simulink model "HITL"  (R2020a)
settings: Solver=ode4  StartTime=0.0  StopTime=100  FixedStep=0.02  RelTol=1e-3  EnableMultiTasking=on
values from neighbouring files (symbols this model uses):
  g = data(5); Quad.b = data(6); Quad.d = data(7); Quad.l = data(8)    [Quad1.m]
undefined symbols (not defined in the file or in its folder): sigbuilder_block
libraries: aerolibutil x10, simulink x9, sharedutil x3, dspindex x2, dspmathops x2, vrlib x1
(part 1 of 2)
settings Model: Creator=Hisham  LastModifiedBy=Hisham
settings DataIOCC: ReturnWorkspaceOutputs=off
settings DebuggingCC: ArithmeticOperatorsInVariantConditions=warning
settings SFSimCC: SimUseLocalCustomCode=off  CustomCodeUndefinedFunction=UseInterfaceOnly
settings RTWCC: RTWUseLocalCustomCode=off
settings CodeAppCC: StateflowObjectComments=on

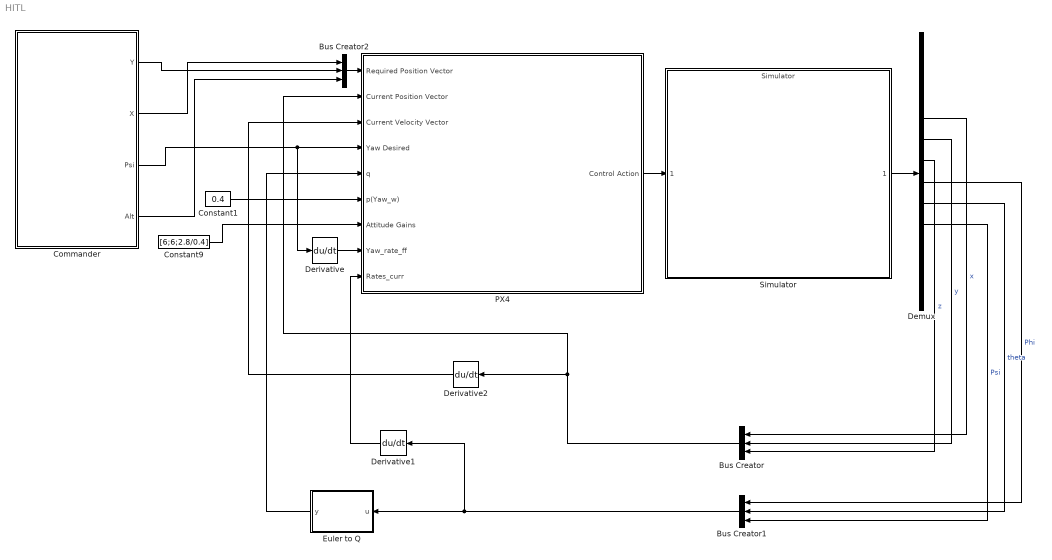
== system HITL ==
  Bus Creator : BusCreator  Inputs=3
  Bus Creator1 : BusCreator  Inputs=3
  Bus Creator2 : BusCreator  Inputs=3
  Commander : Subsystem
  Constant1 : Constant  Value=0.4
  Constant9 : Constant  Value=[6;6;2.8/0.4]
  Demux : Demux  Outputs=12
  Derivative : Derivative
  Derivative1 : Derivative
  Derivative2 : Derivative
  Euler to Q : MATLAB Function  TreatAsAtomicUnit=on
  PX4 : Subsystem
  Simulator : ModelReference  ModelNameDialog=Simulator.slx  SimulationMode=Normal  ModelReferenceVersion=1.27
  wires:
  Commander/2(X) -> Bus Creator2/1
  Commander/3(Psi) -> PX4/4(Yaw Desired), Derivative/1
  Commander/4(Alt) -> Bus Creator2/3
  PX4/1(Control Action) -> Simulator/1
  Demux/8 -> Bus Creator1/2  "theta"
  Demux/5 -> Bus Creator/2  "y"
  Demux/9 -> Bus Creator1/3  "Psi"
  Demux/7 -> Bus Creator1/1  "Phi"
  Demux/4 -> Bus Creator/1  "x"
  Demux/6 -> Bus Creator/3  "z"
  Simulator/1 -> Demux/1
  Bus Creator/1 -> PX4/2(Current Position Vector), Derivative2/1
  Bus Creator1/1 -> Derivative1/1, Euler to Q/1(u)
  Constant1/1 -> PX4/6(p(Yaw_w))
  Constant9/1 -> PX4/7(Attitude Gains)
  Commander/1(Y) -> Bus Creator2/2
  Bus Creator2/1 -> PX4/1(Required Position Vector)
  Derivative/1 -> PX4/8(Yaw_rate_ff)
  Derivative1/1 -> PX4/9(Rates_curr)
  Euler to Q/1(y) -> PX4/5(q)
  Derivative2/1 -> PX4/3(Current Velocity Vector)

== system HITL/Commander ==
  Alt_com : Constant  Value=-3
  Psi_com : Constant  Value=30*2*pi/180
  Signal Builder : Subsystem  Tag=STV Subsys  LoadFcn=sigbuilder_block('load');  StartFcn=sigbuilder_block('start');  StopFcn=sigbuilder_block('stop');  ClipboardFcn=sigbuilder_block('clipboard');  mask(Sigbuilder block){tuvar=[0:10]}
      mask help: Simulink:masks:SigbuilderBlock_MD
      mask init:
      | if ~strcmp(get_param(bdroot(gcbh),'SimulationStatus'),'stopped') tuvar = sigbuilder_block('maskInit'); end
      settings: CopyFcn=sigbuilder_block('copy');  DeleteFcn=sigbuilder_block('delete');  ModelCloseFcn=sigbuilder_block('modelClose');  PreSaveFcn=sigbuilder_block('preSave');  PauseFcn=sigbuilder_block('pause');  ContinueFcn=sigbuilder_block('continue');  NameChangeFcn=sigbuilder_block('namechange');  OpenFcn=sigbuilder_block('open',[6 30 1012.5 447.75 ]);  CloseFcn=sigbuilder_block('close');
      mask Display: plot(0, 0, 100, 100,[2, 2, 32, 32, 2], [68, 8, 8, 68, 68],[32, 2], [38, 38], [32, 19, 2],[53, 60, 44], [32, 17, 17, 2],[16, 16, 31, 31]);txt = getActiveGroup(gcbh);text(2, 100, txt,'verticalAlignment', 'top');
  X_com : Constant  Value=0
  Y_com : Constant  Value=0
  Y : Outport
  X : Outport  Port=2
  Psi : Outport  Port=3
  Alt : Outport  Port=4
  wires:
  Signal Builder/1(Y_com) -> Y/1
  Signal Builder/2(X_com) -> X/1
  Signal Builder/4(psi_com) -> Psi/1
  Signal Builder/3(alt_com) -> Alt/1

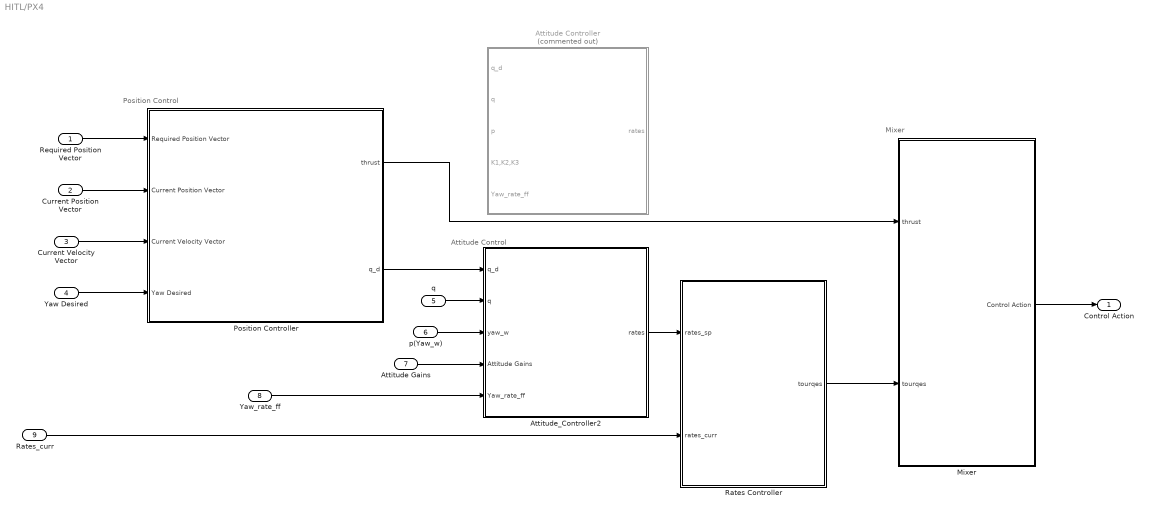
== system HITL/PX4 ==
  note: Mixer
  note: Position Control
  note: Attitude Control
  Required Position Vector : Inport
  Current Position Vector : Inport  Port=2
  Current Velocity Vector : Inport  Port=3
  Yaw Desired : Inport  Port=4
  q : Inport  Port=5
  p(Yaw_w) : Inport  Port=6
  Attitude Gains : Inport  Port=7
  Yaw_rate_ff : Inport  Port=8
  Rates_curr : Inport  Port=9
  Attitude Controller : Subsystem  Commented=on
  Attitude_Controller2 : Subsystem
  Mixer : Subsystem
  Position Controller : Subsystem
  Rates Controller : Subsystem
  Control Action : Outport
  wires:
  Rates_curr/1 -> Rates Controller/2(rates_curr)
  Attitude_Controller2/1(rates) -> Rates Controller/1(rates_sp)
  Mixer/1(Control Action) -> Control Action/1
  Rates Controller/1(tourqes) -> Mixer/2(tourqes)
  q/1 -> Attitude_Controller2/2(q)
  Attitude Gains/1 -> Attitude_Controller2/4(Attitude Gains)
  p(Yaw_w)/1 -> Attitude_Controller2/3(yaw_w)
  Yaw_rate_ff/1 -> Attitude_Controller2/5(Yaw_rate_ff)
  Position Controller/1(thrust) -> Mixer/1(thrust)
  Current Position Vector/1 -> Position Controller/2(Current Position Vector)
  Current Velocity Vector/1 -> Position Controller/3(Current Velocity Vector)
  Required Position Vector/1 -> Position Controller/1(Required Position Vector)
  Yaw Desired/1 -> Position Controller/4(Yaw Desired)
  Position Controller/2(q_d) -> Attitude_Controller2/1(q_d)

== system HITL/Commander/Signal Builder ==
  Demux : Demux  Tag=STV Demux
      settings: DisplayOption=none
  FromWs : FromWorkspace  Tag=STV FromWs  VariableName=tuvar
      SigBuilderData=|
      | common.afterFinalStr = 'Extrapolate'
      | common.sampleTime = 0
      | dataSet.timeRange = [0 60]
      | dataSet.name = 'Group 1'
      | sbobj.Groups.Name = 'Group 1'
      | sbobj.Groups.Signals(1).Name = 'Y_com'
      | sbobj.Groups.Signals(1).XData = [0 4 4 25 25 60]
      | sbobj.Groups.Signals(1).YData = [0 0 5 5 0 0]
      | sbobj.Groups.Signals(2).Name = 'X_com'
      | sbobj.Groups.Signals(2).XData = [0 12 12 42 42 60]
      | sbobj.Groups.Signals(2).YData = [0 0 5 5 0 0]
      | sbobj.Groups.Signals(3).Name = 'alt_com'
      | sbobj.Groups.Signals(3).XData = [0 10 10 60]
      | sbobj.Groups.Signals(3).YData = [1 1 5 5]
      | sbobj.Groups.Signals(4).Name = 'psi_com'
      | sbobj.Groups.Signals(4).XData = [0 1 60]
      | sbobj.Groups.Signals(4).YData = [0 0 0]
      | sbobj.Groups.TimeRange = [0 60]
  Y_com : Outport  Tag=STV Outport
  X_com : Outport  Tag=STV Outport  Port=2
  alt_com : Outport  Tag=STV Outport  Port=3
  psi_com : Outport  Tag=STV Outport  Port=4
  wires:
  FromWs/1 -> Demux/1
  Demux/1 -> Y_com/1
  Demux/2 -> X_com/1
  Demux/3 -> alt_com/1
  Demux/4 -> psi_com/1

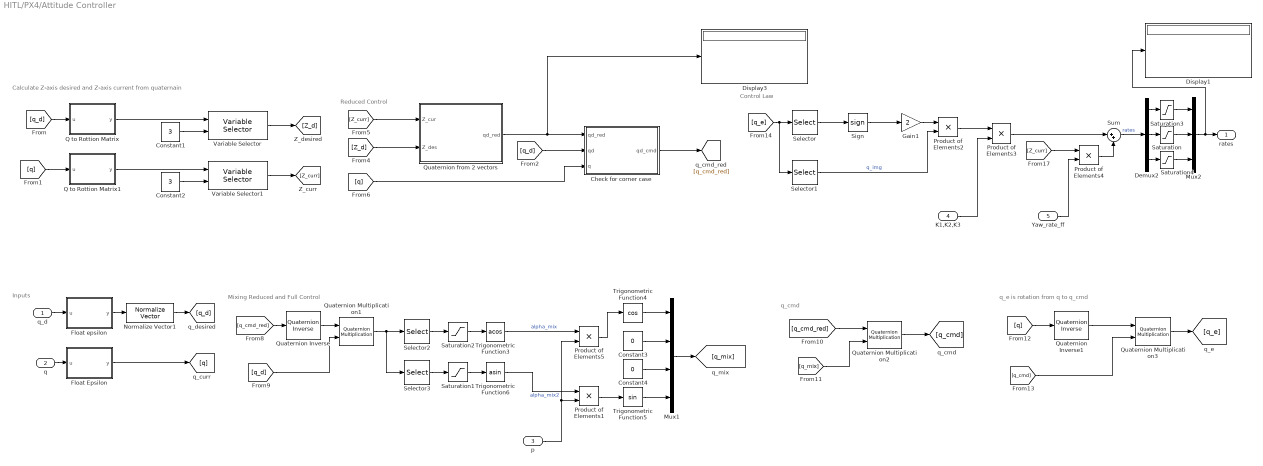
== system HITL/PX4/Attitude Controller ==
  note: Control Law
  note: q_e is rotation from q to q_cmd
  note: Inputs
  note: q_cmd
  note: Mixing Reduced and Full Control
  note: Reduced Control
  note: Calculate Z-axis desired and Z-axis current from quaternain
  q_d : Inport
  q : Inport  Port=2
  p : Inport  Port=3
  K1,K2,K3 : Inport  Port=4
  Yaw_rate_ff : Inport  Port=5
  Check for corner case : MATLAB Function  TreatAsAtomicUnit=on
  Constant1 : Constant  Value=3
  Constant2 : Constant  Value=3
  Constant3 : Constant  Value=0
  Constant4 : Constant  Value=0
  Demux2 : Demux  Outputs=3
  Display1 : Display
  Display3 : Display
  Float Epsilon : MATLAB Function  TreatAsAtomicUnit=on
  Float epsilon : MATLAB Function  TreatAsAtomicUnit=on
  Gain1 : Gain  Gain=2
  Mux1 : Mux
  Mux2 : Mux  Inputs=3
  Normalize Vector1 : vrlib/Utilities/Normalize Vector  maxzero=0
  Product of Elements{1..5} (5 alike) : Product  Inputs=**
  Q to Rottion Matrix : MATLAB Function  TreatAsAtomicUnit=on
  Q to Rottion Matrix1 : MATLAB Function  TreatAsAtomicUnit=on
  Quaternion Inverse : aerolibutil/Quaternion Inverse
  Quaternion Inverse1 : aerolibutil/Quaternion Inverse
  Quaternion Multiplication1 : aerolibutil/Quaternion Multiplication
  Quaternion Multiplication2 : aerolibutil/Quaternion Multiplication
  Quaternion Multiplication3 : aerolibutil/Quaternion Multiplication
  Quaternion from 2 vectors : MATLAB Function  TreatAsAtomicUnit=on
  Saturation : Saturate  UpperLimit=220*pi/180  LowerLimit=-220*pi/180
  Saturation1 : Saturate  UpperLimit=1  LowerLimit=-1
  Saturation2 : Saturate  UpperLimit=1  LowerLimit=-1
  Saturation3 : Saturate  UpperLimit=220*pi/180  LowerLimit=-220*pi/180
  Saturation4 : Saturate  UpperLimit=200*pi/180  LowerLimit=-200*pi/180
  Selector : Selector  InputPortWidth=4  IndexOptions=Index vector (dialog)  Indices=[1]  OutputSizes=1
  Selector1 : Selector  InputPortWidth=4  IndexOptions=Index vector (dialog)  Indices=[2 3 4]  OutputSizes=1
  Selector2 : Selector  InputPortWidth=4  IndexOptions=Index vector (dialog)  Indices=1  OutputSizes=1
  Selector3 : Selector  InputPortWidth=4  IndexOptions=Index vector (dialog)  Indices=4  OutputSizes=1
  Sign : Signum
  Sum : Sum  Inputs=|++
  Trigonometric Function3 : Trigonometry  Operator=acos
  Trigonometric Function4 : Trigonometry  Operator=cos
  Trigonometric Function5 : Trigonometry
  Trigonometric Function6 : Trigonometry  Operator=asin
  Variable Selector : dspindex/Variable Selector  NumInputs=1  rowsOrCols=Columns  IdxMode=Variable  Elements=[1 3]  ZerOneIdxMode=One-based  errmode=Clip Index  FillMode=on  FillValues=0
  Variable Selector1 : dspindex/Variable Selector  NumInputs=1  rowsOrCols=Columns  IdxMode=Variable  Elements=[1 3]  ZerOneIdxMode=One-based  errmode=Clip Index  FillMode=on  FillValues=0
  rates : Outport
  wires:
  Q to Rottion Matrix/1(y) -> Variable Selector/1
  Constant1/1 -> Variable Selector/2
  Q to Rottion Matrix1/1(y) -> Variable Selector1/1
  Constant2/1 -> Variable Selector1/2
  [q_d] -> Q to Rottion Matrix/1(u)
  [q] -> Q to Rottion Matrix1/1(u)
  Variable Selector/1 -> [Z_d]
  Variable Selector1/1 -> [Z_curr]
  [q] -> Check for corner case/3(q)
  Check for corner case/1(qd_cmd) -> [q_cmd_red]
  [q_cmd_red] -> Quaternion Inverse/1
  Quaternion Inverse/1 -> Quaternion Multiplication1/1
  [q_d] -> Quaternion Multiplication1/2
  [q_cmd_red] -> Quaternion Multiplication2/1
  [q_mix] -> Quaternion Multiplication2/2
  Quaternion Multiplication2/1 -> [q_cmd]
  [q] -> Quaternion Inverse1/1
  Quaternion Inverse1/1 -> Quaternion Multiplication3/1
  [q_cmd] -> Quaternion Multiplication3/2
  Quaternion Multiplication3/1 -> [q_e]
  [q_e] -> Selector1/1, Selector/1
  Selector/1 -> Sign/1
  Sign/1 -> Gain1/1
  Gain1/1 -> Product of Elements2/1
  Selector1/1 -> Product of Elements2/2  "q_img"
  Product of Elements2/1 -> Product of Elements3/1
  Product of Elements3/1 -> Sum/1
  [Z_curr] -> Product of Elements4/1
  Product of Elements4/1 -> Sum/2
  Selector2/1 -> Saturation2/1
  Trigonometric Function3/1 -> Product of Elements5/1  "alpha_mix"
  Product of Elements5/1 -> Trigonometric Function4/1
  Trigonometric Function5/1 -> Mux1/4
  Constant4/1 -> Mux1/3
  Constant3/1 -> Mux1/2
  Trigonometric Function4/1 -> Mux1/1
  Mux1/1 -> [q_mix]
  q_d/1 -> Float epsilon/1(u)
  Normalize Vector1/1 -> [q_d]
  Float Epsilon/1(y) -> [q]
  q/1 -> Float Epsilon/1(u)
  Float epsilon/1(y) -> Normalize Vector1/1
  Mux2/1 -> Display1/1, rates/1
  [Z_d] -> Quaternion from 2 vectors/2(Z_des)
  Quaternion from 2 vectors/1(qd_red) -> Display3/1, Check for corner case/1(qd_red)
  [Z_curr] -> Quaternion from 2 vectors/1(Z_cur)
  Demux2/2 -> Saturation/1
  Demux2/3 -> Saturation4/1
  Saturation/1 -> Mux2/2
  Saturation3/1 -> Mux2/1
  Demux2/1 -> Saturation3/1
  Sum/1 -> Demux2/1  "rates"
  Saturation4/1 -> Mux2/3
  [q_d] -> Check for corner case/2(qd)
  Quaternion Multiplication1/1 -> Selector3/1, Selector2/1
  Saturation2/1 -> Trigonometric Function3/1
  K1,K2,K3/1 -> Product of Elements3/2
  Yaw_rate_ff/1 -> Product of Elements4/2
  p/1 -> Product of Elements1/2, Product of Elements5/2
  Saturation1/1 -> Trigonometric Function6/1
  Selector3/1 -> Saturation1/1
  Product of Elements1/1 -> Trigonometric Function5/1
  Trigonometric Function6/1 -> Product of Elements1/1  "alpha_mix2"

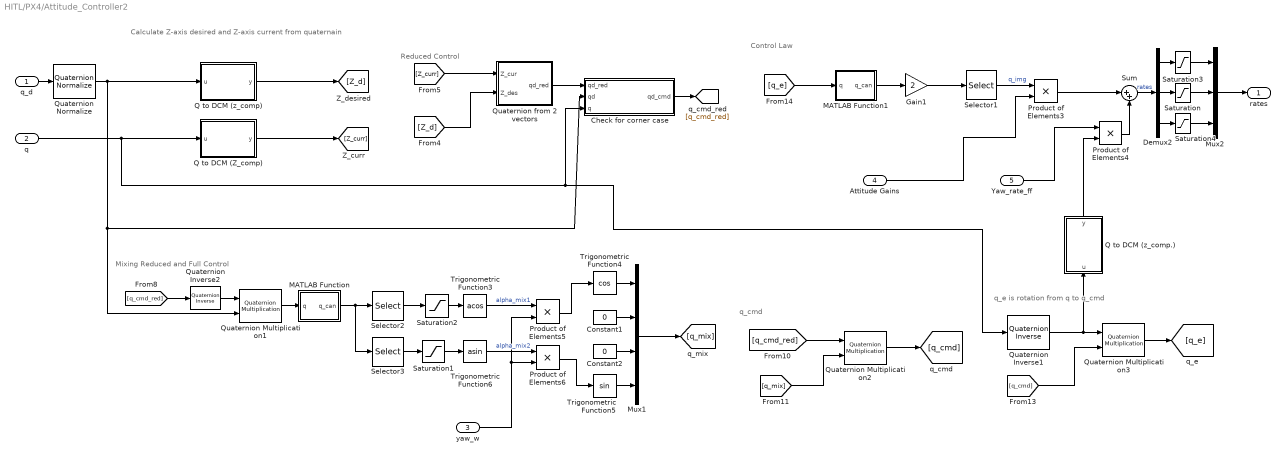
== system HITL/PX4/Attitude_Controller2 ==
  note: Mixing Reduced and Full Control
  note: Calculate Z-axis desired and Z-axis current from quaternain
  note: Control Law
  note: Reduced Control
  note: q_cmd
  note: q_e is rotation from q to q_cmd
  q_d : Inport
  q : Inport  Port=2
  yaw_w : Inport  Port=3
  Attitude Gains : Inport  Port=4
  Yaw_rate_ff : Inport  Port=5
  Check for corner case : MATLAB Function  TreatAsAtomicUnit=on
  Constant1 : Constant  Value=0
  Constant2 : Constant  Value=0
  Demux2 : Demux  Outputs=3
  Gain1 : Gain  Gain=2
  MATLAB Function : MATLAB Function  TreatAsAtomicUnit=on
  MATLAB Function1 : MATLAB Function  TreatAsAtomicUnit=on
  Mux1 : Mux
  Mux2 : Mux  Inputs=3
  Product of Elements{3..6} (4 alike) : Product  Inputs=**
  Q to DCM (Z_comp) : MATLAB Function  TreatAsAtomicUnit=on
  Q to DCM (z_comp) : MATLAB Function  TreatAsAtomicUnit=on
  Q to DCM (z_comp.) : MATLAB Function  TreatAsAtomicUnit=on
  Quaternion Inverse1 : aerolibutil/Quaternion Inverse
  Quaternion Inverse2 : aerolibutil/Quaternion Inverse
  Quaternion Multiplication1 : aerolibutil/Quaternion Multiplication
  Quaternion Multiplication2 : aerolibutil/Quaternion Multiplication
  Quaternion Multiplication3 : aerolibutil/Quaternion Multiplication
  Quaternion Normalize : sharedutil/Quaternion Normalize  aMode=aMode
      settings: SourceProductBaseCode=AE,PW,MT,VE,VP
  Quaternion from 2 vectors : MATLAB Function  TreatAsAtomicUnit=on
  Saturation : Saturate  UpperLimit=220*pi/180  LowerLimit=-220*pi/180
  Saturation1 : Saturate  UpperLimit=1  LowerLimit=-1
  Saturation2 : Saturate  UpperLimit=1  LowerLimit=-1
  Saturation3 : Saturate  UpperLimit=220*pi/180  LowerLimit=-220*pi/180
  Saturation4 : Saturate  UpperLimit=200*pi/180  LowerLimit=-200*pi/180
  Selector1 : Selector  InputPortWidth=4  IndexOptions=Index vector (dialog)  Indices=[2 3 4]  OutputSizes=1
  Selector2 : Selector  InputPortWidth=4  IndexOptions=Index vector (dialog)  Indices=1  OutputSizes=1
  Selector3 : Selector  InputPortWidth=4  IndexOptions=Index vector (dialog)  Indices=4  OutputSizes=1
  Sum : Sum  Inputs=|++
  Trigonometric Function3 : Trigonometry  Operator=acos
  Trigonometric Function4 : Trigonometry  Operator=cos
  Trigonometric Function5 : Trigonometry
  Trigonometric Function6 : Trigonometry  Operator=asin
  rates : Outport
  wires:
  Mux2/1 -> rates/1
  Saturation3/1 -> Mux2/1
  Saturation4/1 -> Mux2/3
  Saturation/1 -> Mux2/2
  Demux2/3 -> Saturation4/1
  Demux2/1 -> Saturation3/1
  Demux2/2 -> Saturation/1
  Sum/1 -> Demux2/1  "rates"
  [Z_d] -> Quaternion from 2 vectors/2(Z_des)
  Quaternion from 2 vectors/1(qd_red) -> Check for corner case/1(qd_red)
  [Z_curr] -> Quaternion from 2 vectors/1(Z_cur)
  MATLAB Function1/1(q_can) -> Gain1/1
  [q_e] -> MATLAB Function1/1(q)
  Gain1/1 -> Selector1/1
  Selector1/1 -> Product of Elements3/1  "q_img"
  Check for corner case/1(qd_cmd) -> [q_cmd_red]
  q/1 -> Q to DCM (Z_comp)/1(u), Quaternion Inverse1/1, Check for corner case/3(q)
  Quaternion Normalize/1 -> Q to DCM (z_comp)/1(u), Check for corner case/2(qd), Quaternion Multiplication1/2
  MATLAB Function/1(q_can) -> Selector2/1, Selector3/1
  Quaternion Multiplication1/1 -> MATLAB Function/1(q)
  q_d/1 -> Quaternion Normalize/1
  Quaternion Inverse2/1 -> Quaternion Multiplication1/1
  [q_cmd_red] -> Quaternion Inverse2/1
  Mux1/1 -> [q_mix]
  Quaternion Inverse1/1 -> Q to DCM (z_comp.)/1(u), Quaternion Multiplication3/1
  Product of Elements3/1 -> Sum/1
  [q_cmd] -> Quaternion Multiplication3/2
  [q_mix] -> Quaternion Multiplication2/2
  [q_cmd_red] -> Quaternion Multiplication2/1
  Selector2/1 -> Saturation2/1
  Quaternion Multiplication3/1 -> [q_e]
  Selector3/1 -> Saturation1/1
  Yaw_rate_ff/1 -> Product of Elements4/1
  Product of Elements4/1 -> Sum/2
  Saturation2/1 -> Trigonometric Function3/1
  Trigonometric Function3/1 -> Product of Elements5/1  "alpha_mix1"
  Quaternion Multiplication2/1 -> [q_cmd]
  Q to DCM (z_comp.)/1(y) -> Product of Elements4/2
  Trigonometric Function4/1 -> Mux1/1
  Product of Elements5/1 -> Trigonometric Function4/1
  Trigonometric Function5/1 -> Mux1/4
  Trigonometric Function6/1 -> Product of Elements6/1  "alpha_mix2"
  Product of Elements6/1 -> Trigonometric Function5/1
  Saturation1/1 -> Trigonometric Function6/1
  Q to DCM (z_comp)/1(y) -> [Z_d]
  Q to DCM (Z_comp)/1(y) -> [Z_curr]
  yaw_w/1 -> Product of Elements5/2, Product of Elements6/2
  Attitude Gains/1 -> Product of Elements3/2
  Constant1/1 -> Mux1/2
  Constant2/1 -> Mux1/3

== system HITL/PX4/Mixer ==
  thrust : Inport
  tourqes : Inport  Port=2
  Display : Display
  "Float Epsilon " : MATLAB Function
  Gain : Gain  Gain=-1
  Iris mixer : Constant  Value=[-0.4377 0.7071 -0.9091 -1; 0.4377 -0.7071 -1 -1; 0.4377 0.7071 0.9091 -1;-0.4377 -0.7071 1 -1]
  Length : MATLABFcn  MATLABFcn=norm
  Mux : Mux  Inputs=2
  Quad_x mixer : Constant  Value=[-0.7071 0.7071 1 -1; 0.7071 -0.7071 1 -1; 0.7071 0.7071 -1 -1;-0.7071 -0.7071 -1 -1]
  Control Action : Outport
  wires:
  thrust/1 -> Length/1
  tourqes/1 -> Mux/1
  Length/1 -> Gain/1
  Mux/1 -> "Float Epsilon "/1(u)
  Gain/1 -> Mux/2
  "Float Epsilon "/1(y) -> Control Action/1, Display/1

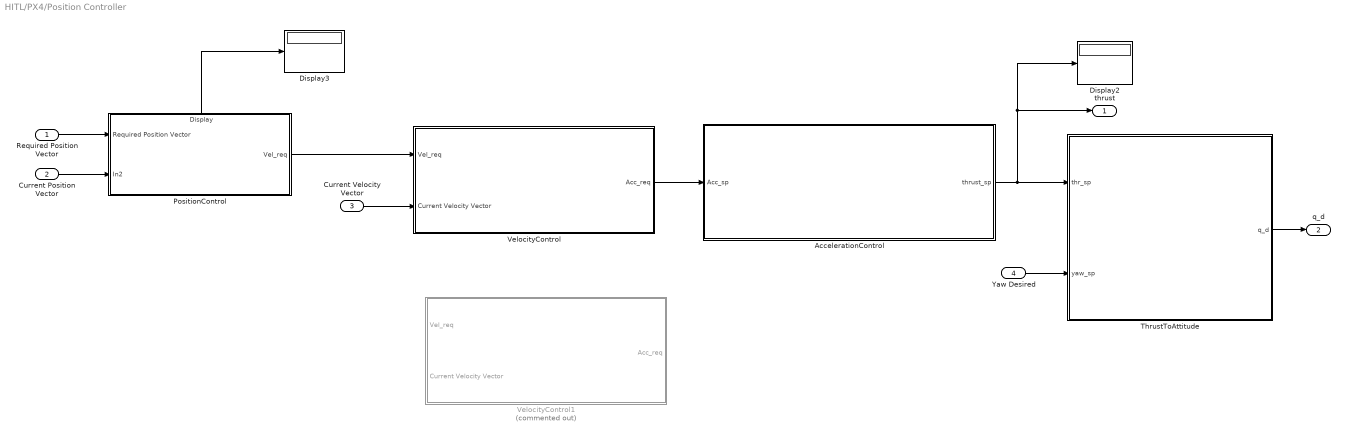
== system HITL/PX4/Position Controller ==
  Required Position Vector : Inport
  Current Position Vector : Inport  Port=2
  Current Velocity Vector : Inport  Port=3
  Yaw Desired : Inport  Port=4
  AccelerationControl : Subsystem
  Display2 : Display
  Display3 : Display
  PositionControl : Subsystem
      settings: PortSchema="{\"entries\":[{\"content\":{\"sides\":[{\"content\":{\"connectorIds\":[\"In1\",\"In2\"]},\"type\":\"ConnectorPlacement.EquallySpacedRectSide\",\"uuid\":\"a4ba3283-86cb-408b-aae8-413f3026a3b7\"},{\"content\":{\"connectorIds\":[\"Out1\"],\"side\":\"RIGHT\"},\"type\":\"ConnectorPlacement.EquallySpacedRectSide\",\"uuid\":\"45b02b29-05a1-4a67-8748-9d19bb26d9bb\"},{\"content\":{\"connectorIds\":[\"Out2\"],\"side\":\"TOP\"},\"type\":\"ConnectorPlacement.EquallySpacedRectSide\",\"uuid\":\"6a5eeb60-33a1-4be7-a33c-7d288ab8de61\"}]},\"type\":\"ConnectorPlacement.EquallySpacedConnector\",\"uuid\":\"25cb5f3a-4277-4784-9d46-e5c601df25b2\"}],\"packageUris\":[\"http://schema.mathworks.com/mf0/Connector/19700101\"],\"version\":\"1.0\"}"
  ThrustToAttitude : Subsystem
  VelocityControl : Subsystem
  VelocityControl1 : Subsystem  Commented=on
  thrust : Outport
  q_d : Outport  Port=2
  wires:
  Required Position Vector/1 -> PositionControl/1(Required Position Vector)
  Current Position Vector/1 -> PositionControl/2(In2)
  PositionControl/2(Display) -> Display3/1
  PositionControl/1(Vel_req) -> VelocityControl/1(Vel_req)
  Current Velocity Vector/1 -> VelocityControl/2(Current Velocity Vector)
  AccelerationControl/1(thrust_sp) -> Display2/1, thrust/1, ThrustToAttitude/1(thr_sp)
  VelocityControl/1(Acc_req) -> AccelerationControl/1(Acc_sp)
  ThrustToAttitude/1(q_d) -> q_d/1
  Yaw Desired/1 -> ThrustToAttitude/2(yaw_sp)

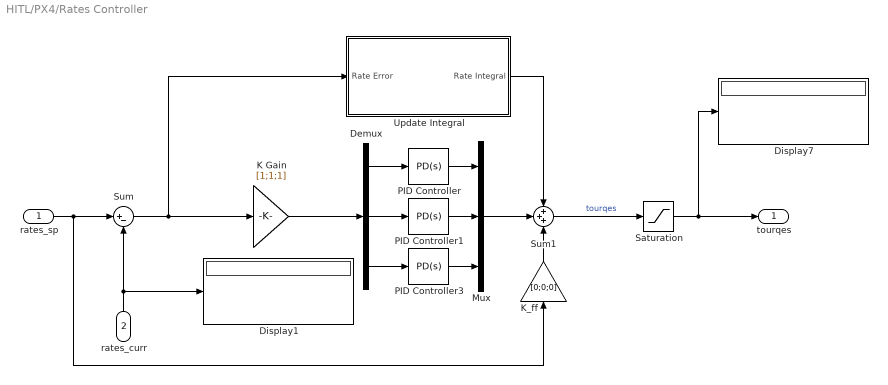
== system HITL/PX4/Rates Controller ==
  rates_sp : Inport
  rates_curr : Inport  Port=2
  Demux : Demux  Outputs=3
  Display1 : Display
  Display7 : Display
  K Gain : Gain  Gain=[1;1;1]
  K_ff : Gain  Gain=[0;0;0]
  Mux : Mux  Inputs=3
  PID Controller : simulink/Continuous/PID Controller  Controller=PD  Form=Parallel  TimeDomain=Continuous-time  UseExternalTs=off  SampleTime=-1  IntegratorMethod=Forward Euler  FilterMethod=Forward Euler  ControllerParametersSource=internal  P=0.2  I=0.2  D=-0.003  UseFilter=on  N=100  TunerSelectOption=Transfer Function Based (PID Tuner App)  InitialConditionSource=internal  InitialConditionForIntegrator=0  InitialConditionForFilter=0  DifferentiatorICPrevScaledInput=0  ExternalReset=none  TrackingMode=off  Kt=1  LimitOutput=off  UpperSaturationLimit=inf  LowerSaturationLimit=-inf  LinearizeAsGain=on  AntiWindupMode=none  Kb=1  POutMin=[]  POutMax=[]  IOutMin=[]  IOutMax=[]  DOutMin=[]  DOutMax=[]  NOutMin=[]  NOutMax=[]  SumOutMin=[]  SumOutMax=[]  SaturationOutMin=[]  SaturationOutMax=[]  PParamMin=[]  PParamMax=[]  IParamMin=[]  IParamMax=[]  DParamMin=[]  DParamMax=[]  NParamMin=[]  NParamMax=[]  KbParamMin=[]  KbParamMax=[]  KtParamMin=[]  KtParamMax=[]  KbOutMin=[]  KbOutMax=[]  KtOutMin=[]  KtOutMax=[]  IntegratorOutMin=[]  IntegratorOutMax=[]  FilterOutMin=[]  FilterOutMax=[]  SumI1OutMin=[]  SumI1OutMax=[]  SumI2OutMin=[]  SumI2OutMax=[]  SumI3OutMin=[]  SumI3OutMax=[]  SumI4OutMin=[]  SumI4OutMax=[]  SumDOutMin=[]  SumDOutMax=[]  DifferentiatorOutMin=[]  DifferentiatorOutMax=[]  FilterDiffOutCoefMin=[]  FilterDiffOutCoefMax=[]  ReciprocalOutMin=[]  ReciprocalOutMax=[]  SumDenOutMin=[]  SumDenOutMax=[]  SumNumOutMin=[]  SumNumOutMax=[]  DivideOutMin=[]  DivideOutMax=[]  UdiffTsProdOutMin=[]  UdiffTsProdOutMax=[]  NTsProdOutMin=[]  NTsProdOutMax=[]  UintegralTsProdOutMin=[]  UintegralTsProdOutMax=[]  UngainTsProdOutMin=[]  UngainTsProdOutMax=[]  IntegratorContinuousStateAttributes=''  IntegratorStateMustResolveToSignalObject=off  IntegratorRTWStateStorageClass=Auto  FilterContinuousStateAttributes=''  FilterStateMustResolveToSignalObject=off  FilterRTWStateStorageClass=Auto  ParallelPVariant=InternalParameters  IdealPVariant=Disabled  IVariant=Disabled  DVariant=InternalParameters  IntegratorVariant=Disabled  SatVariant=Disabled  AWVariant=Disabled  PCopyVariant=Disabled  TRVariant=Disabled  FdbkBlocksVariant=Forward  IdealPFdbkVariant=Disabled  SatFdbkVariant=Disabled  DerivativeFilterVariant=ContFilter  NVariant=InternalParameters  NCopyVariant=Disabled  FilterICVariant=InternalICsFilter  IntegratorICVariant=Disabled  ExternalResetVariant=Disabled  TRSumVariant=Passthrough  SumFdbkVariant=Disabled  SumVariant=Sum_PD  TsampFilterVariant=InternalTs  TsampNgainVariant=Passthrough  TsampIntegralVariant=Disabled_SignalSpec
  PID Controller1 : simulink/Continuous/PID Controller  Controller=PD  Form=Parallel  TimeDomain=Continuous-time  UseExternalTs=off  SampleTime=-1  IntegratorMethod=Forward Euler  FilterMethod=Forward Euler  ControllerParametersSource=internal  P=0.2  I=0.2  D=-0.003  UseFilter=on  N=100  TunerSelectOption=Transfer Function Based (PID Tuner App)  InitialConditionSource=internal  InitialConditionForIntegrator=0  InitialConditionForFilter=0  DifferentiatorICPrevScaledInput=0  ExternalReset=none  TrackingMode=off  Kt=1  LimitOutput=off  UpperSaturationLimit=inf  LowerSaturationLimit=-inf  LinearizeAsGain=on  AntiWindupMode=none  Kb=1  POutMin=[]  POutMax=[]  IOutMin=[]  IOutMax=[]  DOutMin=[]  DOutMax=[]  NOutMin=[]  NOutMax=[]  SumOutMin=[]  SumOutMax=[]  SaturationOutMin=[]  SaturationOutMax=[]  PParamMin=[]  PParamMax=[]  IParamMin=[]  IParamMax=[]  DParamMin=[]  DParamMax=[]  NParamMin=[]  NParamMax=[]  KbParamMin=[]  KbParamMax=[]  KtParamMin=[]  KtParamMax=[]  KbOutMin=[]  KbOutMax=[]  KtOutMin=[]  KtOutMax=[]  IntegratorOutMin=[]  IntegratorOutMax=[]  FilterOutMin=[]  FilterOutMax=[]  SumI1OutMin=[]  SumI1OutMax=[]  SumI2OutMin=[]  SumI2OutMax=[]  SumI3OutMin=[]  SumI3OutMax=[]  SumI4OutMin=[]  SumI4OutMax=[]  SumDOutMin=[]  SumDOutMax=[]  DifferentiatorOutMin=[]  DifferentiatorOutMax=[]  FilterDiffOutCoefMin=[]  FilterDiffOutCoefMax=[]  ReciprocalOutMin=[]  ReciprocalOutMax=[]  SumDenOutMin=[]  SumDenOutMax=[]  SumNumOutMin=[]  SumNumOutMax=[]  DivideOutMin=[]  DivideOutMax=[]  UdiffTsProdOutMin=[]  UdiffTsProdOutMax=[]  NTsProdOutMin=[]  NTsProdOutMax=[]  UintegralTsProdOutMin=[]  UintegralTsProdOutMax=[]  UngainTsProdOutMin=[]  UngainTsProdOutMax=[]  IntegratorContinuousStateAttributes=''  IntegratorStateMustResolveToSignalObject=off  IntegratorRTWStateStorageClass=Auto  FilterContinuousStateAttributes=''  FilterStateMustResolveToSignalObject=off  FilterRTWStateStorageClass=Auto  ParallelPVariant=InternalParameters  IdealPVariant=Disabled  IVariant=Disabled  DVariant=InternalParameters  IntegratorVariant=Disabled  SatVariant=Disabled  AWVariant=Disabled  PCopyVariant=Disabled  TRVariant=Disabled  FdbkBlocksVariant=Forward  IdealPFdbkVariant=Disabled  SatFdbkVariant=Disabled  DerivativeFilterVariant=ContFilter  NVariant=InternalParameters  NCopyVariant=Disabled  FilterICVariant=InternalICsFilter  IntegratorICVariant=Disabled  ExternalResetVariant=Disabled  TRSumVariant=Passthrough  SumFdbkVariant=Disabled  SumVariant=Sum_PD  TsampFilterVariant=InternalTs  TsampNgainVariant=Passthrough  TsampIntegralVariant=Disabled_SignalSpec
  PID Controller3 : simulink/Continuous/PID Controller  Controller=PD  Form=Parallel  TimeDomain=Continuous-time  UseExternalTs=off  SampleTime=-1  IntegratorMethod=Forward Euler  FilterMethod=Forward Euler  ControllerParametersSource=internal  P=0.2  I=0.1  D=0  UseFilter=on  N=100  TunerSelectOption=Transfer Function Based (PID Tuner App)  InitialConditionSource=internal  InitialConditionForIntegrator=0  InitialConditionForFilter=0  DifferentiatorICPrevScaledInput=0  ExternalReset=none  TrackingMode=off  Kt=1  LimitOutput=off  UpperSaturationLimit=inf  LowerSaturationLimit=-inf  LinearizeAsGain=on  AntiWindupMode=none  Kb=1  POutMin=[]  POutMax=[]  IOutMin=[]  IOutMax=[]  DOutMin=[]  DOutMax=[]  NOutMin=[]  NOutMax=[]  SumOutMin=[]  SumOutMax=[]  SaturationOutMin=[]  SaturationOutMax=[]  PParamMin=[]  PParamMax=[]  IParamMin=[]  IParamMax=[]  DParamMin=[]  DParamMax=[]  NParamMin=[]  NParamMax=[]  KbParamMin=[]  KbParamMax=[]  KtParamMin=[]  KtParamMax=[]  KbOutMin=[]  KbOutMax=[]  KtOutMin=[]  KtOutMax=[]  IntegratorOutMin=[]  IntegratorOutMax=[]  FilterOutMin=[]  FilterOutMax=[]  SumI1OutMin=[]  SumI1OutMax=[]  SumI2OutMin=[]  SumI2OutMax=[]  SumI3OutMin=[]  SumI3OutMax=[]  SumI4OutMin=[]  SumI4OutMax=[]  SumDOutMin=[]  SumDOutMax=[]  DifferentiatorOutMin=[]  DifferentiatorOutMax=[]  FilterDiffOutCoefMin=[]  FilterDiffOutCoefMax=[]  ReciprocalOutMin=[]  ReciprocalOutMax=[]  SumDenOutMin=[]  SumDenOutMax=[]  SumNumOutMin=[]  SumNumOutMax=[]  DivideOutMin=[]  DivideOutMax=[]  UdiffTsProdOutMin=[]  UdiffTsProdOutMax=[]  NTsProdOutMin=[]  NTsProdOutMax=[]  UintegralTsProdOutMin=[]  UintegralTsProdOutMax=[]  UngainTsProdOutMin=[]  UngainTsProdOutMax=[]  IntegratorContinuousStateAttributes=''  IntegratorStateMustResolveToSignalObject=off  IntegratorRTWStateStorageClass=Auto  FilterContinuousStateAttributes=''  FilterStateMustResolveToSignalObject=off  FilterRTWStateStorageClass=Auto  ParallelPVariant=InternalParameters  IdealPVariant=Disabled  IVariant=Disabled  DVariant=InternalParameters  IntegratorVariant=Disabled  SatVariant=Disabled  AWVariant=Disabled  PCopyVariant=Disabled  TRVariant=Disabled  FdbkBlocksVariant=Forward  IdealPFdbkVariant=Disabled  SatFdbkVariant=Disabled  DerivativeFilterVariant=ContFilter  NVariant=InternalParameters  NCopyVariant=Disabled  FilterICVariant=InternalICsFilter  IntegratorICVariant=Disabled  ExternalResetVariant=Disabled  TRSumVariant=Passthrough  SumFdbkVariant=Disabled  SumVariant=Sum_PD  TsampFilterVariant=InternalTs  TsampNgainVariant=Passthrough  TsampIntegralVariant=Disabled_SignalSpec
  Saturation : Saturate  UpperLimit=1  LowerLimit=-1
  Sum : Sum  Inputs=|+-
  Sum1 : Sum  Inputs=+++
  Update Integral : Subsystem
  tourqes : Outport
  wires:
  Sum1/1 -> Saturation/1  "tourqes"
  Sum/1 -> Update Integral/1(Rate Error), K Gain/1
  Demux/3 -> PID Controller3/1
  Demux/2 -> PID Controller1/1
  Demux/1 -> PID Controller/1
  PID Controller1/1 -> Mux/2
  PID Controller/1 -> Mux/1
  Saturation/1 -> Display7/1, tourqes/1
  PID Controller3/1 -> Mux/3
  K Gain/1 -> Demux/1
  rates_sp/1 -> K_ff/1, Sum/1
  Mux/1 -> Sum1/2
  K_ff/1 -> Sum1/3
  Update Integral/1(Rate Integral) -> Sum1/1
  rates_curr/1 -> Display1/1, Sum/2

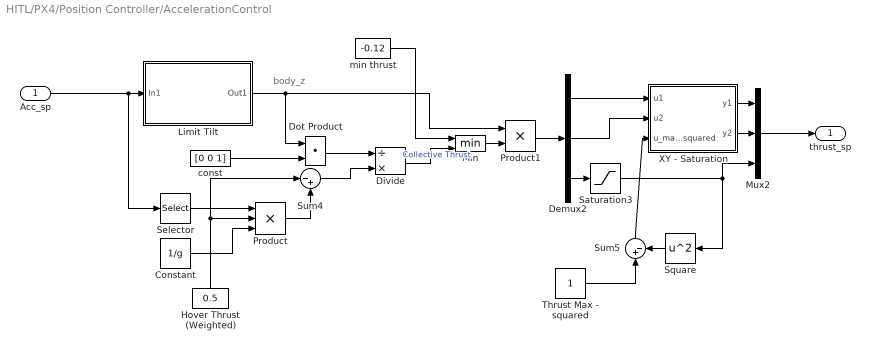
== system HITL/PX4/Position Controller/AccelerationControl ==
  note: body_z
  Acc_sp : Inport
  Constant : Constant  Value=1/g
  Demux2 : Demux  Outputs=3
  Divide : Product  Inputs=/*
  Dot Product : DotProduct  InputSameDT=on  OutDataTypeStr=Inherit: Inherit via internal rule
  Hover Thrust (Weighted) : Constant  Value=0.5
  Limit Tilt : Subsystem
  Min : MinMax  Inputs=2
  Mux2 : Mux  Inputs=3
  Product : Product  Inputs=3
  Product1 : Product
  Saturation3 : Saturate  UpperLimit=0  LowerLimit=-1
  Selector : Selector  InputPortWidth=3  IndexOptions=Index vector (dialog)  Indices=[3]  OutputSizes=1
  Square : Math  Operator=square  SaturateOnIntegerOverflow=on
  Sum4 : Sum  Inputs=|-+
  Sum5 : Sum  Inputs=|+-
  Thrust Max - squared : Constant
  XY - Saturation : MATLAB Function  TreatAsAtomicUnit=on
  const : Constant  Value=[0 0 1]
  min thrust : Constant  Value=-0.12
  thrust_sp : Outport
  wires:
  Limit Tilt/1(Out1) -> Product1/1, Dot Product/1
  Selector/1 -> Product/1
  Acc_sp/1 -> Selector/1, Limit Tilt/1(In1)
  Square/1 -> Sum5/2
  Saturation3/1 -> Mux2/3, Square/1
  Demux2/2 -> XY - Saturation/2(u2)
  Constant/1 -> Product/3
  XY - Saturation/2(y2) -> Mux2/2
  Hover Thrust (Weighted)/1 -> Product/2, Sum4/1
  XY - Saturation/1(y1) -> Mux2/1
  Demux2/1 -> XY - Saturation/1(u1)
  Demux2/3 -> Saturation3/1
  min thrust/1 -> Min/1
  Dot Product/1 -> Divide/1
  Product/1 -> Sum4/2
  const/1 -> Dot Product/2
  Product1/1 -> Demux2/1
  Sum4/1 -> Divide/2
  Min/1 -> Product1/2
  Thrust Max - squared/1 -> Sum5/1
  Divide/1 -> Min/2  "Collective Thrust"
  Sum5/1 -> XY - Saturation/3(u_max_squared)
  Mux2/1 -> thrust_sp/1

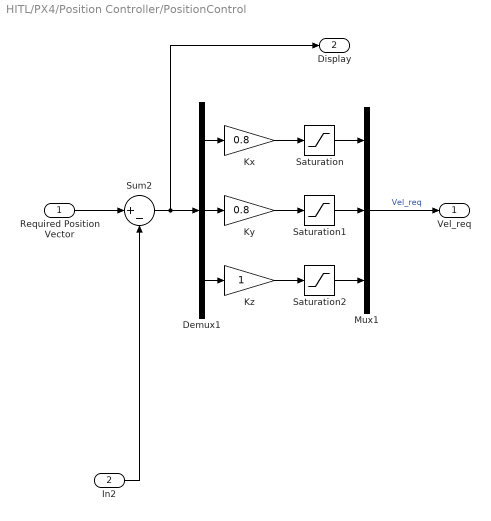
== system HITL/PX4/Position Controller/PositionControl ==
  Required Position Vector : Inport
  In2 : Inport  Port=2
  Demux1 : Demux  Outputs=3
  Kx : Gain  Gain=0.8
  Ky : Gain  Gain=0.8
  Kz : Gain
  Mux1 : Mux  Inputs=3
  Saturation : Saturate  UpperLimit=12  LowerLimit=-12
  Saturation1 : Saturate  UpperLimit=12  LowerLimit=-12
  Saturation2 : Saturate  UpperLimit=1  LowerLimit=-3
  Sum2 : Sum  Inputs=|+-
  Vel_req : Outport
  Display : Outport  Port=2
  wires:
  Demux1/3 -> Kz/1
  Demux1/2 -> Ky/1
  Saturation1/1 -> Mux1/2
  Kx/1 -> Saturation/1
  Required Position Vector/1 -> Sum2/1
  Demux1/1 -> Kx/1
  Saturation/1 -> Mux1/1
  Ky/1 -> Saturation1/1
  Sum2/1 -> Display/1, Demux1/1
  Saturation2/1 -> Mux1/3
  Kz/1 -> Saturation2/1
  In2/1 -> Sum2/2
  Mux1/1 -> Vel_req/1  "Vel_req"

== system HITL/PX4/Position Controller/ThrustToAttitude ==
  thr_sp : Inport
  yaw_sp : Inport  Port=2
  Matrix Concatenate : Concatenate  NumInputs=3  Mode=Multidimensional array  ConcatenateDimension=2
  Rotaion Matrix To Q : MATLAB Function  TreatAsAtomicUnit=on
  Thrust To Attitude : Subsystem
  q_d : Outport
  wires:
  Thrust To Attitude/3(Rz) -> Matrix Concatenate/3
  Matrix Concatenate/1 -> Rotaion Matrix To Q/1(u)  "R_sp"
  Thrust To Attitude/1(Rx) -> Matrix Concatenate/1
  Thrust To Attitude/2(Ry) -> Matrix Concatenate/2
  Rotaion Matrix To Q/1(y) -> q_d/1  "q_d"
  thr_sp/1 -> Thrust To Attitude/1(thr_sp)
  yaw_sp/1 -> Thrust To Attitude/2(yaw_sp)

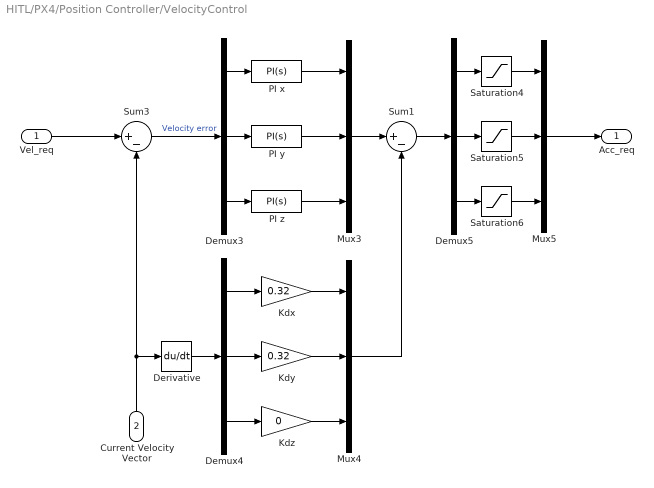
== system HITL/PX4/Position Controller/VelocityControl ==
  Vel_req : Inport
  Current Velocity Vector : Inport  Port=2
  Demux3 : Demux  Outputs=3
  Demux4 : Demux  Outputs=3
  Demux5 : Demux  Outputs=3
  Derivative : Derivative
  Kdx : Gain  Gain=0.32
  Kdy : Gain  Gain=0.32
  Kdz : Gain  Gain=0
  Mux3 : Mux  Inputs=3
  Mux4 : Mux  Inputs=3
  Mux5 : Mux  Inputs=3
  PI x : simulink/Continuous/PID Controller  Controller=PI  Form=Parallel  TimeDomain=Continuous-time  UseExternalTs=off  SampleTime=-1  IntegratorMethod=Forward Euler  FilterMethod=Forward Euler  ControllerParametersSource=internal  P=4  I=0.4  D=-0.32  UseFilter=on  N=100  TunerSelectOption=Transfer Function Based (PID Tuner App)  InitialConditionSource=internal  InitialConditionForIntegrator=0  InitialConditionForFilter=0  DifferentiatorICPrevScaledInput=0  ExternalReset=none  TrackingMode=off  Kt=1  LimitOutput=off  UpperSaturationLimit=5  LowerSaturationLimit=-5  LinearizeAsGain=on  AntiWindupMode=none  Kb=1  POutMin=[]  POutMax=[]  IOutMin=[]  IOutMax=[]  DOutMin=[]  DOutMax=[]  NOutMin=[]  NOutMax=[]  SumOutMin=[]  SumOutMax=[]  SaturationOutMin=[]  SaturationOutMax=[]  PParamMin=[]  PParamMax=[]  IParamMin=[]  IParamMax=[]  DParamMin=[]  DParamMax=[]  NParamMin=[]  NParamMax=[]  KbParamMin=[]  KbParamMax=[]  KtParamMin=[]  KtParamMax=[]  KbOutMin=[]  KbOutMax=[]  KtOutMin=[]  KtOutMax=[]  IntegratorOutMin=[]  IntegratorOutMax=[]  FilterOutMin=[]  FilterOutMax=[]  SumI1OutMin=[]  SumI1OutMax=[]  SumI2OutMin=[]  SumI2OutMax=[]  SumI3OutMin=[]  SumI3OutMax=[]  SumI4OutMin=[]  SumI4OutMax=[]  SumDOutMin=[]  SumDOutMax=[]  DifferentiatorOutMin=[]  DifferentiatorOutMax=[]  FilterDiffOutCoefMin=[]  FilterDiffOutCoefMax=[]  ReciprocalOutMin=[]  ReciprocalOutMax=[]  SumDenOutMin=[]  SumDenOutMax=[]  SumNumOutMin=[]  SumNumOutMax=[]  DivideOutMin=[]  DivideOutMax=[]  UdiffTsProdOutMin=[]  UdiffTsProdOutMax=[]  NTsProdOutMin=[]  NTsProdOutMax=[]  UintegralTsProdOutMin=[]  UintegralTsProdOutMax=[]  UngainTsProdOutMin=[]  UngainTsProdOutMax=[]  IntegratorContinuousStateAttributes=''  IntegratorStateMustResolveToSignalObject=off  IntegratorRTWStateStorageClass=Auto  FilterContinuousStateAttributes=''  FilterStateMustResolveToSignalObject=off  FilterRTWStateStorageClass=Auto  ParallelPVariant=InternalParameters  IdealPVariant=Disabled  IVariant=InternalParameters  DVariant=Disabled  IntegratorVariant=Continuous  SatVariant=Disabled  AWVariant=Passthrough  PCopyVariant=Disabled  TRVariant=Disabled  FdbkBlocksVariant=Forward  IdealPFdbkVariant=Disabled  SatFdbkVariant=Disabled  DerivativeFilterVariant=Disabled  NVariant=Disabled  NCopyVariant=Disabled_SignalSpec  FilterICVariant=Disabled  IntegratorICVariant=InternalICs  ExternalResetVariant=Disabled  TRSumVariant=Passthrough  SumFdbkVariant=Disabled  SumVariant=Sum_PI  TsampFilterVariant=InternalTs  TsampNgainVariant=Passthrough  TsampIntegralVariant=Passthrough
  PI y : simulink/Continuous/PID Controller  Controller=PI  Form=Parallel  TimeDomain=Continuous-time  UseExternalTs=off  SampleTime=-1  IntegratorMethod=Forward Euler  FilterMethod=Forward Euler  ControllerParametersSource=internal  P=4  I=0.4  D=-0.32  UseFilter=on  N=100  TunerSelectOption=Transfer Function Based (PID Tuner App)  InitialConditionSource=internal  InitialConditionForIntegrator=0  InitialConditionForFilter=0  DifferentiatorICPrevScaledInput=0  ExternalReset=none  TrackingMode=off  Kt=1  LimitOutput=off  UpperSaturationLimit=5  LowerSaturationLimit=-5  LinearizeAsGain=on  AntiWindupMode=none  Kb=1  POutMin=[]  POutMax=[]  IOutMin=[]  IOutMax=[]  DOutMin=[]  DOutMax=[]  NOutMin=[]  NOutMax=[]  SumOutMin=[]  SumOutMax=[]  SaturationOutMin=[]  SaturationOutMax=[]  PParamMin=[]  PParamMax=[]  IParamMin=[]  IParamMax=[]  DParamMin=[]  DParamMax=[]  NParamMin=[]  NParamMax=[]  KbParamMin=[]  KbParamMax=[]  KtParamMin=[]  KtParamMax=[]  KbOutMin=[]  KbOutMax=[]  KtOutMin=[]  KtOutMax=[]  IntegratorOutMin=[]  IntegratorOutMax=[]  FilterOutMin=[]  FilterOutMax=[]  SumI1OutMin=[]  SumI1OutMax=[]  SumI2OutMin=[]  SumI2OutMax=[]  SumI3OutMin=[]  SumI3OutMax=[]  SumI4OutMin=[]  SumI4OutMax=[]  SumDOutMin=[]  SumDOutMax=[]  DifferentiatorOutMin=[]  DifferentiatorOutMax=[]  FilterDiffOutCoefMin=[]  FilterDiffOutCoefMax=[]  ReciprocalOutMin=[]  ReciprocalOutMax=[]  SumDenOutMin=[]  SumDenOutMax=[]  SumNumOutMin=[]  SumNumOutMax=[]  DivideOutMin=[]  DivideOutMax=[]  UdiffTsProdOutMin=[]  UdiffTsProdOutMax=[]  NTsProdOutMin=[]  NTsProdOutMax=[]  UintegralTsProdOutMin=[]  UintegralTsProdOutMax=[]  UngainTsProdOutMin=[]  UngainTsProdOutMax=[]  IntegratorContinuousStateAttributes=''  IntegratorStateMustResolveToSignalObject=off  IntegratorRTWStateStorageClass=Auto  FilterContinuousStateAttributes=''  FilterStateMustResolveToSignalObject=off  FilterRTWStateStorageClass=Auto  ParallelPVariant=InternalParameters  IdealPVariant=Disabled  IVariant=InternalParameters  DVariant=Disabled  IntegratorVariant=Continuous  SatVariant=Disabled  AWVariant=Passthrough  PCopyVariant=Disabled  TRVariant=Disabled  FdbkBlocksVariant=Forward  IdealPFdbkVariant=Disabled  SatFdbkVariant=Disabled  DerivativeFilterVariant=Disabled  NVariant=Disabled  NCopyVariant=Disabled_SignalSpec  FilterICVariant=Disabled  IntegratorICVariant=InternalICs  ExternalResetVariant=Disabled  TRSumVariant=Passthrough  SumFdbkVariant=Disabled  SumVariant=Sum_PI  TsampFilterVariant=InternalTs  TsampNgainVariant=Passthrough  TsampIntegralVariant=Passthrough
  PI z : simulink/Continuous/PID Controller  Controller=PI  Form=Parallel  TimeDomain=Continuous-time  UseExternalTs=off  SampleTime=-1  IntegratorMethod=Forward Euler  FilterMethod=Forward Euler  ControllerParametersSource=internal  P=12  I=3  D=0  UseFilter=on  N=100  TunerSelectOption=Transfer Function Based (PID Tuner App)  InitialConditionSource=internal  InitialConditionForIntegrator=0  InitialConditionForFilter=0  DifferentiatorICPrevScaledInput=0  ExternalReset=none  TrackingMode=off  Kt=1  LimitOutput=off  UpperSaturationLimit=3  LowerSaturationLimit=-4  LinearizeAsGain=on  AntiWindupMode=none  Kb=1  POutMin=[]  POutMax=[]  IOutMin=[]  IOutMax=[]  DOutMin=[]  DOutMax=[]  NOutMin=[]  NOutMax=[]  SumOutMin=[]  SumOutMax=[]  SaturationOutMin=[]  SaturationOutMax=[]  PParamMin=[]  PParamMax=[]  IParamMin=[]  IParamMax=[]  DParamMin=[]  DParamMax=[]  NParamMin=[]  NParamMax=[]  KbParamMin=[]  KbParamMax=[]  KtParamMin=[]  KtParamMax=[]  KbOutMin=[]  KbOutMax=[]  KtOutMin=[]  KtOutMax=[]  IntegratorOutMin=[]  IntegratorOutMax=[]  FilterOutMin=[]  FilterOutMax=[]  SumI1OutMin=[]  SumI1OutMax=[]  SumI2OutMin=[]  SumI2OutMax=[]  SumI3OutMin=[]  SumI3OutMax=[]  SumI4OutMin=[]  SumI4OutMax=[]  SumDOutMin=[]  SumDOutMax=[]  DifferentiatorOutMin=[]  DifferentiatorOutMax=[]  FilterDiffOutCoefMin=[]  FilterDiffOutCoefMax=[]  ReciprocalOutMin=[]  ReciprocalOutMax=[]  SumDenOutMin=[]  SumDenOutMax=[]  SumNumOutMin=[]  SumNumOutMax=[]  DivideOutMin=[]  DivideOutMax=[]  UdiffTsProdOutMin=[]  UdiffTsProdOutMax=[]  NTsProdOutMin=[]  NTsProdOutMax=[]  UintegralTsProdOutMin=[]  UintegralTsProdOutMax=[]  UngainTsProdOutMin=[]  UngainTsProdOutMax=[]  IntegratorContinuousStateAttributes=''  IntegratorStateMustResolveToSignalObject=off  IntegratorRTWStateStorageClass=Auto  FilterContinuousStateAttributes=''  FilterStateMustResolveToSignalObject=off  FilterRTWStateStorageClass=Auto  ParallelPVariant=InternalParameters  IdealPVariant=Disabled  IVariant=InternalParameters  DVariant=Disabled  IntegratorVariant=Continuous  SatVariant=Disabled  AWVariant=Passthrough  PCopyVariant=Disabled  TRVariant=Disabled  FdbkBlocksVariant=Forward  IdealPFdbkVariant=Disabled  SatFdbkVariant=Disabled  DerivativeFilterVariant=Disabled  NVariant=Disabled  NCopyVariant=Disabled_SignalSpec  FilterICVariant=Disabled  IntegratorICVariant=InternalICs  ExternalResetVariant=Disabled  TRSumVariant=Passthrough  SumFdbkVariant=Disabled  SumVariant=Sum_PI  TsampFilterVariant=InternalTs  TsampNgainVariant=Passthrough  TsampIntegralVariant=Passthrough
  Saturation4 : Saturate  UpperLimit=5  LowerLimit=-5
  Saturation5 : Saturate  UpperLimit=5  LowerLimit=-5
  Saturation6 : Saturate  UpperLimit=3  LowerLimit=-4
  Sum1 : Sum  Inputs=|+-
  Sum3 : Sum  Inputs=|+-
  Acc_req : Outport
  wires:
  Demux3/1 -> PI x/1
  Kdy/1 -> Mux4/2
  Demux3/2 -> PI y/1
  Demux5/3 -> Saturation6/1
  Sum3/1 -> Demux3/1  "Velocity error"
  Sum1/1 -> Demux5/1
  PI x/1 -> Mux3/1
  Demux5/1 -> Saturation4/1
  Kdx/1 -> Mux4/1
  Demux3/3 -> PI z/1
  Saturation5/1 -> Mux5/2
  Derivative/1 -> Demux4/1
  Saturation4/1 -> Mux5/1
  PI z/1 -> Mux3/3
  Demux5/2 -> Saturation5/1
  Demux4/2 -> Kdy/1
  Mux4/1 -> Sum1/2
  Saturation6/1 -> Mux5/3
  Mux5/1 -> Acc_req/1
  Demux4/1 -> Kdx/1
  Mux3/1 -> Sum1/1
  Current Velocity Vector/1 -> Sum3/2, Derivative/1
  PI y/1 -> Mux3/2
  Demux4/3 -> Kdz/1
  Kdz/1 -> Mux4/3
  Vel_req/1 -> Sum3/1

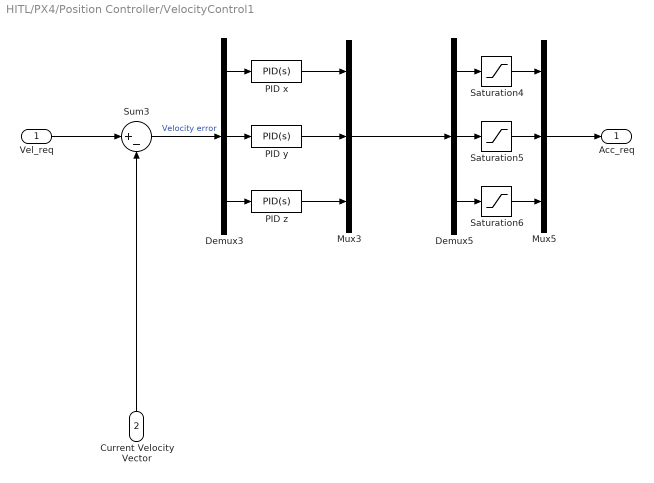
== system HITL/PX4/Position Controller/VelocityControl1 ==
  Vel_req : Inport
  Current Velocity Vector : Inport  Port=2
  Demux3 : Demux  Outputs=3
  Demux5 : Demux  Outputs=3
  Mux3 : Mux  Inputs=3
  Mux5 : Mux  Inputs=3
  PID x : simulink/Continuous/PID Controller  Controller=PID  Form=Parallel  TimeDomain=Continuous-time  UseExternalTs=off  SampleTime=-1  IntegratorMethod=Forward Euler  FilterMethod=Forward Euler  ControllerParametersSource=internal  P=4  I=0.4  D=-0.32  UseFilter=on  N=100  TunerSelectOption=Transfer Function Based (PID Tuner App)  InitialConditionSource=internal  InitialConditionForIntegrator=0  InitialConditionForFilter=0  DifferentiatorICPrevScaledInput=0  ExternalReset=none  TrackingMode=off  Kt=1  LimitOutput=off  UpperSaturationLimit=5  LowerSaturationLimit=-5  LinearizeAsGain=on  AntiWindupMode=none  Kb=1  POutMin=[]  POutMax=[]  IOutMin=[]  IOutMax=[]  DOutMin=[]  DOutMax=[]  NOutMin=[]  NOutMax=[]  SumOutMin=[]  SumOutMax=[]  SaturationOutMin=[]  SaturationOutMax=[]  PParamMin=[]  PParamMax=[]  IParamMin=[]  IParamMax=[]  DParamMin=[]  DParamMax=[]  NParamMin=[]  NParamMax=[]  KbParamMin=[]  KbParamMax=[]  KtParamMin=[]  KtParamMax=[]  KbOutMin=[]  KbOutMax=[]  KtOutMin=[]  KtOutMax=[]  IntegratorOutMin=[]  IntegratorOutMax=[]  FilterOutMin=[]  FilterOutMax=[]  SumI1OutMin=[]  SumI1OutMax=[]  SumI2OutMin=[]  SumI2OutMax=[]  SumI3OutMin=[]  SumI3OutMax=[]  SumI4OutMin=[]  SumI4OutMax=[]  SumDOutMin=[]  SumDOutMax=[]  DifferentiatorOutMin=[]  DifferentiatorOutMax=[]  FilterDiffOutCoefMin=[]  FilterDiffOutCoefMax=[]  ReciprocalOutMin=[]  ReciprocalOutMax=[]  SumDenOutMin=[]  SumDenOutMax=[]  SumNumOutMin=[]  SumNumOutMax=[]  DivideOutMin=[]  DivideOutMax=[]  UdiffTsProdOutMin=[]  UdiffTsProdOutMax=[]  NTsProdOutMin=[]  NTsProdOutMax=[]  UintegralTsProdOutMin=[]  UintegralTsProdOutMax=[]  UngainTsProdOutMin=[]  UngainTsProdOutMax=[]  IntegratorContinuousStateAttributes=''  IntegratorStateMustResolveToSignalObject=off  IntegratorRTWStateStorageClass=Auto  FilterContinuousStateAttributes=''  FilterStateMustResolveToSignalObject=off  FilterRTWStateStorageClass=Auto  ParallelPVariant=InternalParameters  IdealPVariant=Disabled  IVariant=InternalParameters  DVariant=InternalParameters  IntegratorVariant=Continuous  SatVariant=Disabled  AWVariant=Passthrough  PCopyVariant=Disabled  TRVariant=Disabled  FdbkBlocksVariant=Forward  IdealPFdbkVariant=Disabled  SatFdbkVariant=Disabled  DerivativeFilterVariant=ContFilter  NVariant=InternalParameters  NCopyVariant=Disabled  FilterICVariant=InternalICsFilter  IntegratorICVariant=InternalICs  ExternalResetVariant=Disabled  TRSumVariant=Passthrough  SumFdbkVariant=Disabled  SumVariant=Sum_PID  TsampFilterVariant=InternalTs  TsampNgainVariant=Passthrough  TsampIntegralVariant=Passthrough
  PID y : simulink/Continuous/PID Controller  Controller=PID  Form=Parallel  TimeDomain=Continuous-time  UseExternalTs=off  SampleTime=-1  IntegratorMethod=Forward Euler  FilterMethod=Forward Euler  ControllerParametersSource=internal  P=4  I=0.4  D=-0.32  UseFilter=on  N=100  TunerSelectOption=Transfer Function Based (PID Tuner App)  InitialConditionSource=internal  InitialConditionForIntegrator=0  InitialConditionForFilter=0  DifferentiatorICPrevScaledInput=0  ExternalReset=none  TrackingMode=off  Kt=1  LimitOutput=off  UpperSaturationLimit=5  LowerSaturationLimit=-5  LinearizeAsGain=on  AntiWindupMode=none  Kb=1  POutMin=[]  POutMax=[]  IOutMin=[]  IOutMax=[]  DOutMin=[]  DOutMax=[]  NOutMin=[]  NOutMax=[]  SumOutMin=[]  SumOutMax=[]  SaturationOutMin=[]  SaturationOutMax=[]  PParamMin=[]  PParamMax=[]  IParamMin=[]  IParamMax=[]  DParamMin=[]  DParamMax=[]  NParamMin=[]  NParamMax=[]  KbParamMin=[]  KbParamMax=[]  KtParamMin=[]  KtParamMax=[]  KbOutMin=[]  KbOutMax=[]  KtOutMin=[]  KtOutMax=[]  IntegratorOutMin=[]  IntegratorOutMax=[]  FilterOutMin=[]  FilterOutMax=[]  SumI1OutMin=[]  SumI1OutMax=[]  SumI2OutMin=[]  SumI2OutMax=[]  SumI3OutMin=[]  SumI3OutMax=[]  SumI4OutMin=[]  SumI4OutMax=[]  SumDOutMin=[]  SumDOutMax=[]  DifferentiatorOutMin=[]  DifferentiatorOutMax=[]  FilterDiffOutCoefMin=[]  FilterDiffOutCoefMax=[]  ReciprocalOutMin=[]  ReciprocalOutMax=[]  SumDenOutMin=[]  SumDenOutMax=[]  SumNumOutMin=[]  SumNumOutMax=[]  DivideOutMin=[]  DivideOutMax=[]  UdiffTsProdOutMin=[]  UdiffTsProdOutMax=[]  NTsProdOutMin=[]  NTsProdOutMax=[]  UintegralTsProdOutMin=[]  UintegralTsProdOutMax=[]  UngainTsProdOutMin=[]  UngainTsProdOutMax=[]  IntegratorContinuousStateAttributes=''  IntegratorStateMustResolveToSignalObject=off  IntegratorRTWStateStorageClass=Auto  FilterContinuousStateAttributes=''  FilterStateMustResolveToSignalObject=off  FilterRTWStateStorageClass=Auto  ParallelPVariant=InternalParameters  IdealPVariant=Disabled  IVariant=InternalParameters  DVariant=InternalParameters  IntegratorVariant=Continuous  SatVariant=Disabled  AWVariant=Passthrough  PCopyVariant=Disabled  TRVariant=Disabled  FdbkBlocksVariant=Forward  IdealPFdbkVariant=Disabled  SatFdbkVariant=Disabled  DerivativeFilterVariant=ContFilter  NVariant=InternalParameters  NCopyVariant=Disabled  FilterICVariant=InternalICsFilter  IntegratorICVariant=InternalICs  ExternalResetVariant=Disabled  TRSumVariant=Passthrough  SumFdbkVariant=Disabled  SumVariant=Sum_PID  TsampFilterVariant=InternalTs  TsampNgainVariant=Passthrough  TsampIntegralVariant=Passthrough
  PID z : simulink/Continuous/PID Controller  Controller=PID  Form=Parallel  TimeDomain=Continuous-time  UseExternalTs=off  SampleTime=-1  IntegratorMethod=Forward Euler  FilterMethod=Forward Euler  ControllerParametersSource=internal  P=12  I=3  D=0  UseFilter=on  N=100  TunerSelectOption=Transfer Function Based (PID Tuner App)  InitialConditionSource=internal  InitialConditionForIntegrator=0  InitialConditionForFilter=0  DifferentiatorICPrevScaledInput=0  ExternalReset=none  TrackingMode=off  Kt=1  LimitOutput=off  UpperSaturationLimit=3  LowerSaturationLimit=-4  LinearizeAsGain=on  AntiWindupMode=none  Kb=1  POutMin=[]  POutMax=[]  IOutMin=[]  IOutMax=[]  DOutMin=[]  DOutMax=[]  NOutMin=[]  NOutMax=[]  SumOutMin=[]  SumOutMax=[]  SaturationOutMin=[]  SaturationOutMax=[]  PParamMin=[]  PParamMax=[]  IParamMin=[]  IParamMax=[]  DParamMin=[]  DParamMax=[]  NParamMin=[]  NParamMax=[]  KbParamMin=[]  KbParamMax=[]  KtParamMin=[]  KtParamMax=[]  KbOutMin=[]  KbOutMax=[]  KtOutMin=[]  KtOutMax=[]  IntegratorOutMin=[]  IntegratorOutMax=[]  FilterOutMin=[]  FilterOutMax=[]  SumI1OutMin=[]  SumI1OutMax=[]  SumI2OutMin=[]  SumI2OutMax=[]  SumI3OutMin=[]  SumI3OutMax=[]  SumI4OutMin=[]  SumI4OutMax=[]  SumDOutMin=[]  SumDOutMax=[]  DifferentiatorOutMin=[]  DifferentiatorOutMax=[]  FilterDiffOutCoefMin=[]  FilterDiffOutCoefMax=[]  ReciprocalOutMin=[]  ReciprocalOutMax=[]  SumDenOutMin=[]  SumDenOutMax=[]  SumNumOutMin=[]  SumNumOutMax=[]  DivideOutMin=[]  DivideOutMax=[]  UdiffTsProdOutMin=[]  UdiffTsProdOutMax=[]  NTsProdOutMin=[]  NTsProdOutMax=[]  UintegralTsProdOutMin=[]  UintegralTsProdOutMax=[]  UngainTsProdOutMin=[]  UngainTsProdOutMax=[]  IntegratorContinuousStateAttributes=''  IntegratorStateMustResolveToSignalObject=off  IntegratorRTWStateStorageClass=Auto  FilterContinuousStateAttributes=''  FilterStateMustResolveToSignalObject=off  FilterRTWStateStorageClass=Auto  ParallelPVariant=InternalParameters  IdealPVariant=Disabled  IVariant=InternalParameters  DVariant=InternalParameters  IntegratorVariant=Continuous  SatVariant=Disabled  AWVariant=Passthrough  PCopyVariant=Disabled  TRVariant=Disabled  FdbkBlocksVariant=Forward  IdealPFdbkVariant=Disabled  SatFdbkVariant=Disabled  DerivativeFilterVariant=ContFilter  NVariant=InternalParameters  NCopyVariant=Disabled  FilterICVariant=InternalICsFilter  IntegratorICVariant=InternalICs  ExternalResetVariant=Disabled  TRSumVariant=Passthrough  SumFdbkVariant=Disabled  SumVariant=Sum_PID  TsampFilterVariant=InternalTs  TsampNgainVariant=Passthrough  TsampIntegralVariant=Passthrough
  Saturation4 : Saturate  UpperLimit=5  LowerLimit=-5
  Saturation5 : Saturate  UpperLimit=5  LowerLimit=-5
  Saturation6 : Saturate  UpperLimit=3  LowerLimit=-4
  Sum3 : Sum  Inputs=|+-
  Acc_req : Outport
  wires:
  Demux3/1 -> PID x/1
  Demux3/2 -> PID y/1
  Demux5/3 -> Saturation6/1
  Sum3/1 -> Demux3/1  "Velocity error"
  Mux3/1 -> Demux5/1
  PID x/1 -> Mux3/1
  Demux5/1 -> Saturation4/1
  Demux3/3 -> PID z/1
  Saturation5/1 -> Mux5/2
  Saturation4/1 -> Mux5/1
  PID z/1 -> Mux3/3
  Demux5/2 -> Saturation5/1
  Saturation6/1 -> Mux5/3
  Mux5/1 -> Acc_req/1
  Current Velocity Vector/1 -> Sum3/2
  PID y/1 -> Mux3/2
  Vel_req/1 -> Sum3/1

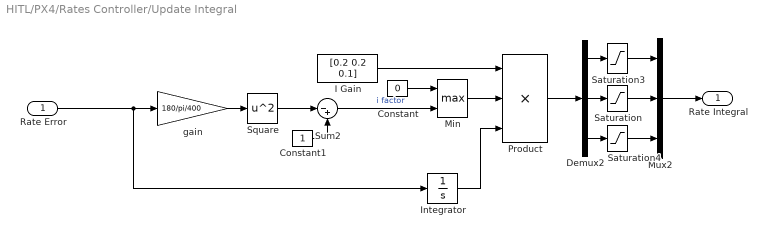
== system HITL/PX4/Rates Controller/Update Integral ==
  Rate Error : Inport
  Constant : Constant  Value=0
  Constant1 : Constant
  Demux2 : Demux  Outputs=3
  I Gain : Constant  Value=[0.2 0.2 0.1]
  Integrator : Integrator
  Min : MinMax  Function=max  Inputs=2
  Mux2 : Mux  Inputs=3
  Product : Product  Inputs=3
  Saturation : Saturate  UpperLimit=0.3  LowerLimit=-0.3
  Saturation3 : Saturate  UpperLimit=0.3  LowerLimit=-0.3
  Saturation4 : Saturate  UpperLimit=0.3  LowerLimit=-0.3
  Square : Math  Operator=square  SaturateOnIntegerOverflow=on
  Sum2 : Sum  Inputs=|-+
  gain : Gain  Gain=180/pi/400
  Rate Integral : Outport
  wires:
  Constant1/1 -> Sum2/2
  Rate Error/1 -> Integrator/1, gain/1
  Square/1 -> Sum2/1
  Min/1 -> Product/2
  Constant/1 -> Min/1
  Sum2/1 -> Min/2  "i factor"
  Integrator/1 -> Product/3
  gain/1 -> Square/1
  I Gain/1 -> Product/1
  Mux2/1 -> Rate Integral/1
  Demux2/2 -> Saturation/1
  Saturation4/1 -> Mux2/3
  Demux2/3 -> Saturation4/1
  Saturation/1 -> Mux2/2
  Saturation3/1 -> Mux2/1
  Demux2/1 -> Saturation3/1
  Product/1 -> Demux2/1
